simulink model "ur10_NN_v1"  (R2022b)
settings: Solver=ode4  StartTime=0.0  StopTime=5  FixedStep=0.01  MaxStep=0.1  RelTol=1e-2  AbsTol=1e-2
model workspace (MAT data in the model file):
  jointLimits = [-2.94087978961 -2.50454747661 -2.94087978961 -2.15548162621 -5.06145483078 -1.53588974176 -3.99680398707 0 0 -2.94087978961 -2.50454747661 -2.94087978961 ... (36 elements, 18x2)]
  q_points = [-0.521158884693  0.491931392418; -0.226045107026  -0.192139666701; -0.000470673510356  -0.00321781893086; 0.204187486975  0.0825184830426; -0.516935337839  0.505690245866; 0.0199734933983  0.0998802945608]
undefined symbols (not defined in the file): cbf_parms, obstacle, replay_rate, ur10
libraries: robotmaniplib x29, neural x27, robotcorelib x10
(part 2 of 2)

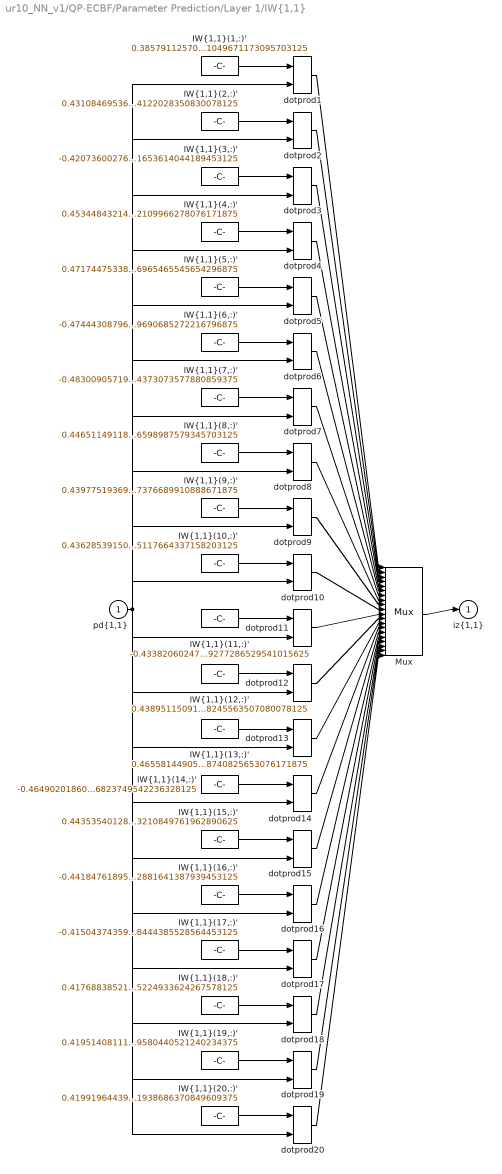
== system ur10_NN_v1/QP-ECBF/Parameter Prediction/Layer 1/IW{1,1} ==
  "pd{1,1}" : Inport  PortDimensions=1
      mask Display: e = 0.06;c1 = [120 230 180]/255;c2 = ([120 230 180]+0)/(256+128);c3 = ([120 230 180]+128)/(256+128);patch([0 1 1 0],[0 0 1 1],c1);patch([0 1 1 1-e 1-e 0+e],[0 0 1 1-e 0+e 0+e],c2);patch([0 0 1 1-e 0+e 0+e],[0 1 1 1-e 1-e 0+e],c3);plot([0 1 1 0 0],[0 0 1 1 0]);
  "IW{1,1}(1,:)'" : Constant  Value=0.385791125708176363406920472698402591049671173095703125
      mask Display: e = 0.06;c1 = [120 150 230]/255;c2 = ([120 150 230]+0)/383;c3 = ([120 150 230]+128)/383;patch([0 1 1 0],[0 0 1 1],c1);patch([0 1 1 1-e 1-e 0+e],[0 0 1 1-e 0+e 0+e],c2);patch([0 0 1 1-e 0+e 0+e],[0 1 1 1-e 1-e 0+e],c3);plot([0 1 1 0 0],[0 0 1 1 0]);disp('Weights');
  "IW{1,1}(10,:)'" : Constant  Value=0.43628539150201117724492405614000745117664337158203125
      mask Display: e = 0.06;c1 = [120 150 230]/255;c2 = ([120 150 230]+0)/383;c3 = ([120 150 230]+128)/383;patch([0 1 1 0],[0 0 1 1],c1);patch([0 1 1 1-e 1-e 0+e],[0 0 1 1-e 0+e 0+e],c2);patch([0 0 1 1-e 0+e 0+e],[0 1 1 1-e 1-e 0+e],c3);plot([0 1 1 0 0],[0 0 1 1 0]);disp('Weights');
  "IW{1,1}(11,:)'" : Constant  Value=-0.433820602471342964268075093059451319277286529541015625
      mask Display: e = 0.06;c1 = [120 150 230]/255;c2 = ([120 150 230]+0)/383;c3 = ([120 150 230]+128)/383;patch([0 1 1 0],[0 0 1 1],c1);patch([0 1 1 1-e 1-e 0+e],[0 0 1 1-e 0+e 0+e],c2);patch([0 0 1 1-e 0+e 0+e],[0 1 1 1-e 1-e 0+e],c3);plot([0 1 1 0 0],[0 0 1 1 0]);disp('Weights');
  "IW{1,1}(12,:)'" : Constant  Value=0.438951150918765187203263167248223908245563507080078125
      mask Display: e = 0.06;c1 = [120 150 230]/255;c2 = ([120 150 230]+0)/383;c3 = ([120 150 230]+128)/383;patch([0 1 1 0],[0 0 1 1],c1);patch([0 1 1 1-e 1-e 0+e],[0 0 1 1-e 0+e 0+e],c2);patch([0 0 1 1-e 0+e 0+e],[0 1 1 1-e 1-e 0+e],c3);plot([0 1 1 0 0],[0 0 1 1 0]);disp('Weights');
  "IW{1,1}(13,:)'" : Constant  Value=0.465581449051758411439294604861061088740825653076171875
      mask Display: e = 0.06;c1 = [120 150 230]/255;c2 = ([120 150 230]+0)/383;c3 = ([120 150 230]+128)/383;patch([0 1 1 0],[0 0 1 1],c1);patch([0 1 1 1-e 1-e 0+e],[0 0 1 1-e 0+e 0+e],c2);patch([0 0 1 1-e 0+e 0+e],[0 1 1 1-e 1-e 0+e],c3);plot([0 1 1 0 0],[0 0 1 1 0]);disp('Weights');
  "IW{1,1}(14,:)'" : Constant  Value=-0.464902018604204159135662166590918786823749542236328125
      mask Display: e = 0.06;c1 = [120 150 230]/255;c2 = ([120 150 230]+0)/383;c3 = ([120 150 230]+128)/383;patch([0 1 1 0],[0 0 1 1],c1);patch([0 1 1 1-e 1-e 0+e],[0 0 1 1-e 0+e 0+e],c2);patch([0 0 1 1-e 0+e 0+e],[0 1 1 1-e 1-e 0+e],c3);plot([0 1 1 0 0],[0 0 1 1 0]);disp('Weights');
  "IW{1,1}(15,:)'" : Constant  Value=0.44353540128859325619714581989683210849761962890625
      mask Display: e = 0.06;c1 = [120 150 230]/255;c2 = ([120 150 230]+0)/383;c3 = ([120 150 230]+128)/383;patch([0 1 1 0],[0 0 1 1],c1);patch([0 1 1 1-e 1-e 0+e],[0 0 1 1-e 0+e 0+e],c2);patch([0 0 1 1-e 0+e 0+e],[0 1 1 1-e 1-e 0+e],c3);plot([0 1 1 0 0],[0 0 1 1 0]);disp('Weights');
  "IW{1,1}(16,:)'" : Constant  Value=-0.441847618958016330470428556509432382881641387939453125
      mask Display: e = 0.06;c1 = [120 150 230]/255;c2 = ([120 150 230]+0)/383;c3 = ([120 150 230]+128)/383;patch([0 1 1 0],[0 0 1 1],c1);patch([0 1 1 1-e 1-e 0+e],[0 0 1 1-e 0+e 0+e],c2);patch([0 0 1 1-e 0+e 0+e],[0 1 1 1-e 1-e 0+e],c3);plot([0 1 1 0 0],[0 0 1 1 0]);disp('Weights');
  "IW{1,1}(17,:)'" : Constant  Value=-0.41504374359596785115655848130700178444385528564453125
      mask Display: e = 0.06;c1 = [120 150 230]/255;c2 = ([120 150 230]+0)/383;c3 = ([120 150 230]+128)/383;patch([0 1 1 0],[0 0 1 1],c1);patch([0 1 1 1-e 1-e 0+e],[0 0 1 1-e 0+e 0+e],c2);patch([0 0 1 1-e 0+e 0+e],[0 1 1 1-e 1-e 0+e],c3);plot([0 1 1 0 0],[0 0 1 1 0]);disp('Weights');
  "IW{1,1}(18,:)'" : Constant  Value=0.417688385219415814209042991933529265224933624267578125
      mask Display: e = 0.06;c1 = [120 150 230]/255;c2 = ([120 150 230]+0)/383;c3 = ([120 150 230]+128)/383;patch([0 1 1 0],[0 0 1 1],c1);patch([0 1 1 1-e 1-e 0+e],[0 0 1 1-e 0+e 0+e],c2);patch([0 0 1 1-e 0+e 0+e],[0 1 1 1-e 1-e 0+e],c3);plot([0 1 1 0 0],[0 0 1 1 0]);disp('Weights');
  "IW{1,1}(19,:)'" : Constant  Value=0.41951408111363386321812640744610689580440521240234375
      mask Display: e = 0.06;c1 = [120 150 230]/255;c2 = ([120 150 230]+0)/383;c3 = ([120 150 230]+128)/383;patch([0 1 1 0],[0 0 1 1],c1);patch([0 1 1 1-e 1-e 0+e],[0 0 1 1-e 0+e 0+e],c2);patch([0 0 1 1-e 0+e 0+e],[0 1 1 1-e 1-e 0+e],c3);plot([0 1 1 0 0],[0 0 1 1 0]);disp('Weights');
  "IW{1,1}(2,:)'" : Constant  Value=0.431084695364223613456289285750244744122028350830078125
      mask Display: e = 0.06;c1 = [120 150 230]/255;c2 = ([120 150 230]+0)/383;c3 = ([120 150 230]+128)/383;patch([0 1 1 0],[0 0 1 1],c1);patch([0 1 1 1-e 1-e 0+e],[0 0 1 1-e 0+e 0+e],c2);patch([0 0 1 1-e 0+e 0+e],[0 1 1 1-e 1-e 0+e],c3);plot([0 1 1 0 0],[0 0 1 1 0]);disp('Weights');
  "IW{1,1}(20,:)'" : Constant  Value=0.41991964439801332531487787491641938686370849609375
      mask Display: e = 0.06;c1 = [120 150 230]/255;c2 = ([120 150 230]+0)/383;c3 = ([120 150 230]+128)/383;patch([0 1 1 0],[0 0 1 1],c1);patch([0 1 1 1-e 1-e 0+e],[0 0 1 1-e 0+e 0+e],c2);patch([0 0 1 1-e 0+e 0+e],[0 1 1 1-e 1-e 0+e],c3);plot([0 1 1 0 0],[0 0 1 1 0]);disp('Weights');
  "IW{1,1}(3,:)'" : Constant  Value=-0.4207360027662521151370356164989061653614044189453125
      mask Display: e = 0.06;c1 = [120 150 230]/255;c2 = ([120 150 230]+0)/383;c3 = ([120 150 230]+128)/383;patch([0 1 1 0],[0 0 1 1],c1);patch([0 1 1 1-e 1-e 0+e],[0 0 1 1-e 0+e 0+e],c2);patch([0 0 1 1-e 0+e 0+e],[0 1 1 1-e 1-e 0+e],c3);plot([0 1 1 0 0],[0 0 1 1 0]);disp('Weights');
  "IW{1,1}(4,:)'" : Constant  Value=0.4534484321497032066616839074413292109966278076171875
      mask Display: e = 0.06;c1 = [120 150 230]/255;c2 = ([120 150 230]+0)/383;c3 = ([120 150 230]+128)/383;patch([0 1 1 0],[0 0 1 1],c1);patch([0 1 1 1-e 1-e 0+e],[0 0 1 1-e 0+e 0+e],c2);patch([0 0 1 1-e 0+e 0+e],[0 1 1 1-e 1-e 0+e],c3);plot([0 1 1 0 0],[0 0 1 1 0]);disp('Weights');
  "IW{1,1}(5,:)'" : Constant  Value=0.471744753381412695869556728212046436965465545654296875
      mask Display: e = 0.06;c1 = [120 150 230]/255;c2 = ([120 150 230]+0)/383;c3 = ([120 150 230]+128)/383;patch([0 1 1 0],[0 0 1 1],c1);patch([0 1 1 1-e 1-e 0+e],[0 0 1 1-e 0+e 0+e],c2);patch([0 0 1 1-e 0+e 0+e],[0 1 1 1-e 1-e 0+e],c3);plot([0 1 1 0 0],[0 0 1 1 0]);disp('Weights');
  "IW{1,1}(6,:)'" : Constant  Value=-0.474443087961794407458882005812483839690685272216796875
      mask Display: e = 0.06;c1 = [120 150 230]/255;c2 = ([120 150 230]+0)/383;c3 = ([120 150 230]+128)/383;patch([0 1 1 0],[0 0 1 1],c1);patch([0 1 1 1-e 1-e 0+e],[0 0 1 1-e 0+e 0+e],c2);patch([0 0 1 1-e 0+e 0+e],[0 1 1 1-e 1-e 0+e],c3);plot([0 1 1 0 0],[0 0 1 1 0]);disp('Weights');
  "IW{1,1}(7,:)'" : Constant  Value=-0.483009057197872238020863733254373073577880859375
      mask Display: e = 0.06;c1 = [120 150 230]/255;c2 = ([120 150 230]+0)/383;c3 = ([120 150 230]+128)/383;patch([0 1 1 0],[0 0 1 1],c1);patch([0 1 1 1-e 1-e 0+e],[0 0 1 1-e 0+e 0+e],c2);patch([0 0 1 1-e 0+e 0+e],[0 1 1 1-e 1-e 0+e],c3);plot([0 1 1 0 0],[0 0 1 1 0]);disp('Weights');
  "IW{1,1}(8,:)'" : Constant  Value=0.446511491183943232119446520300698466598987579345703125
      mask Display: e = 0.06;c1 = [120 150 230]/255;c2 = ([120 150 230]+0)/383;c3 = ([120 150 230]+128)/383;patch([0 1 1 0],[0 0 1 1],c1);patch([0 1 1 1-e 1-e 0+e],[0 0 1 1-e 0+e 0+e],c2);patch([0 0 1 1-e 0+e 0+e],[0 1 1 1-e 1-e 0+e],c3);plot([0 1 1 0 0],[0 0 1 1 0]);disp('Weights');
  "IW{1,1}(9,:)'" : Constant  Value=0.4397751936978948616996376586030237376689910888671875
      mask Display: e = 0.06;c1 = [120 150 230]/255;c2 = ([120 150 230]+0)/383;c3 = ([120 150 230]+128)/383;patch([0 1 1 0],[0 0 1 1],c1);patch([0 1 1 1-e 1-e 0+e],[0 0 1 1-e 0+e 0+e],c2);patch([0 0 1 1-e 0+e 0+e],[0 1 1 1-e 1-e 0+e],c3);plot([0 1 1 0 0],[0 0 1 1 0]);disp('Weights');
  Mux : Mux  Inputs=20
      mask Display: e = 0.06;c1 = [120 150 230]/255;c2 = ([120 150 230]+0)/383;c3 = ([120 150 230]+128)/383;patch([0 1 1 0],[0 0 1 1],c1);patch([0 1 1 1-e 1-e 0+e],[0 0 1 1-e 0+e 0+e],c2);patch([0 0 1 1-e 0+e 0+e],[0 1 1 1-e 1-e 0+e],c3);plot([0 1 1 0 0],[0 0 1 1 0]);disp('Mux');
  dotprod{1..20} (20 alike) : neural/Weight Functions/dotprod
  "iz{1,1}" : Outport
      mask Display: e = 0.06;c1 = [120 230 180]/255;c2 = ([120 230 180]+0)/(256+128);c3 = ([120 230 180]+128)/(256+128);patch([0 1 1 0],[0 0 1 1],c1);patch([0 1 1 1-e 1-e 0+e],[0 0 1 1-e 0+e 0+e],c2);patch([0 0 1 1-e 0+e 0+e],[0 1 1 1-e 1-e 0+e],c3);plot([0 1 1 0 0],[0 0 1 1 0]);
  wires:
  "IW{1,1}(1,:)'"/1 -> dotprod1/1
  "pd{1,1}"/1 -> dotprod1/2, dotprod2/2, dotprod3/2, dotprod4/2, dotprod5/2, dotprod6/2, dotprod7/2, dotprod8/2, dotprod9/2, dotprod10/2, dotprod11/2, dotprod12/2, dotprod13/2, dotprod14/2, dotprod15/2, dotprod16/2, dotprod17/2, dotprod18/2, dotprod19/2, dotprod20/2
  dotprod1/1 -> Mux/1
  "IW{1,1}(2,:)'"/1 -> dotprod2/1
  dotprod2/1 -> Mux/2
  "IW{1,1}(3,:)'"/1 -> dotprod3/1
  dotprod3/1 -> Mux/3
  "IW{1,1}(4,:)'"/1 -> dotprod4/1
  dotprod4/1 -> Mux/4
  "IW{1,1}(5,:)'"/1 -> dotprod5/1
  dotprod5/1 -> Mux/5
  "IW{1,1}(6,:)'"/1 -> dotprod6/1
  dotprod6/1 -> Mux/6
  "IW{1,1}(7,:)'"/1 -> dotprod7/1
  dotprod7/1 -> Mux/7
  "IW{1,1}(8,:)'"/1 -> dotprod8/1
  dotprod8/1 -> Mux/8
  "IW{1,1}(9,:)'"/1 -> dotprod9/1
  dotprod9/1 -> Mux/9
  "IW{1,1}(10,:)'"/1 -> dotprod10/1
  dotprod10/1 -> Mux/10
  "IW{1,1}(11,:)'"/1 -> dotprod11/1
  dotprod11/1 -> Mux/11
  "IW{1,1}(12,:)'"/1 -> dotprod12/1
  dotprod12/1 -> Mux/12
  "IW{1,1}(13,:)'"/1 -> dotprod13/1
  dotprod13/1 -> Mux/13
  "IW{1,1}(14,:)'"/1 -> dotprod14/1
  dotprod14/1 -> Mux/14
  "IW{1,1}(15,:)'"/1 -> dotprod15/1
  dotprod15/1 -> Mux/15
  "IW{1,1}(16,:)'"/1 -> dotprod16/1
  dotprod16/1 -> Mux/16
  "IW{1,1}(17,:)'"/1 -> dotprod17/1
  dotprod17/1 -> Mux/17
  "IW{1,1}(18,:)'"/1 -> dotprod18/1
  dotprod18/1 -> Mux/18
  "IW{1,1}(19,:)'"/1 -> dotprod19/1
  dotprod19/1 -> Mux/19
  "IW{1,1}(20,:)'"/1 -> dotprod20/1
  dotprod20/1 -> Mux/20
  Mux/1 -> "iz{1,1}"/1

== system ur10_NN_v1/QP-ECBF/Parameter Prediction/Layer 2/Delays 1 ==
  "p{2}" : Inport  PortDimensions=20
      mask Display: e = 0.06;c1 = [120 230 180]/255;c2 = ([120 230 180]+0)/(256+128);c3 = ([120 230 180]+128)/(256+128);patch([0 1 1 0],[0 0 1 1],c1);patch([0 1 1 1-e 1-e 0+e],[0 0 1 1-e 0+e 0+e],c2);patch([0 0 1 1-e 0+e 0+e],[0 1 1 1-e 1-e 0+e],c3);plot([0 1 1 0 0],[0 0 1 1 0]);
  mux : Mux  Inputs=1
      mask Display: e = 0.06;c1 = [120 150 230]/255;c2 = ([120 150 230]+0)/383;c3 = ([120 150 230]+128)/383;patch([0 1 1 0],[0 0 1 1],c1);patch([0 1 1 1-e 1-e 0+e],[0 0 1 1-e 0+e 0+e],c2);patch([0 0 1 1-e 0+e 0+e],[0 1 1 1-e 1-e 0+e],c3);plot([0 1 1 0 0],[0 0 1 1 0]);disp('Mux')
  "pd{2,1}" : Outport
      mask Display: e = 0.06;c1 = [120 230 180]/255;c2 = ([120 230 180]+0)/(256+128);c3 = ([120 230 180]+128)/(256+128);patch([0 1 1 0],[0 0 1 1],c1);patch([0 1 1 1-e 1-e 0+e],[0 0 1 1-e 0+e 0+e],c2);patch([0 0 1 1-e 0+e 0+e],[0 1 1 1-e 1-e 0+e],c3);plot([0 1 1 0 0],[0 0 1 1 0]);
  wires:
  "p{2}"/1 -> mux/1
  mux/1 -> "pd{2,1}"/1

== system ur10_NN_v1/QP-ECBF/Parameter Prediction/Layer 2/LW{2,1} ==
  "ad{2,1}" : Inport  PortDimensions=20
      mask Display: e = 0.06;c1 = [120 230 180]/255;c2 = ([120 230 180]+0)/(256+128);c3 = ([120 230 180]+128)/(256+128);patch([0 1 1 0],[0 0 1 1],c1);patch([0 1 1 1-e 1-e 0+e],[0 0 1 1-e 0+e 0+e],c2);patch([0 0 1 1-e 0+e 0+e],[0 1 1 1-e 1-e 0+e],c3);plot([0 1 1 0 0],[0 0 1 1 0]);
  "IW{2,1}(1,:)'" : Constant  Value=[-0.1626878657231537184113534522111876867711544036865234375;-0.1200341041433554689632501322194002568721771240234375;0.1005644547301407787376348323959973640739917755126953125;-0.0218554638658896051295332796371440053917467594146728515625;0.046984730038880005709156506554791121743619441986083984375;-0.06521551214731112489086939376647933386266231536865234375;-0.09351088155010280067447325791363255120813846588134765625;0.054747137380286116370431415134589769877493381500244140625;0.035620000191153682045364092800809885375201702117919921875;0.00647129243408957333105746556611848063766956329345703125;0.0304926056112096548200707246678575756959617137908935546875;-0.032706609699335316421286989907457609660923480987548828125;-0.03896160134336344726957435113945393823087215423583984375;0.0120722770013152007340107019217612105421721935272216796875;0.0089858125649034288617844623558994499035179615020751953125;-0.0185507146410883345943876321371135418303310871124267578125;-0.01055971666121561895745895043319251271896064281463623046875;0.0011611856964841254895304256677945886622183024883270263671875;0.021181318555724769348014291381332441233098506927490234375;0.0093270870010835615904198903081123717129230499267578125]
      mask Display: e = 0.06;c1 = [120 150 230]/255;c2 = ([120 150 230]+0)/383;c3 = ([120 150 230]+128)/383;patch([0 1 1 0],[0 0 1 1],c1);patch([0 1 1 1-e 1-e 0+e],[0 0 1 1-e 0+e 0+e],c2);patch([0 0 1 1-e 0+e 0+e],[0 1 1 1-e 1-e 0+e],c3);plot([0 1 1 0 0],[0 0 1 1 0]);disp('weights');
  "IW{2,1}(2,:)'" : Constant  Value=[0.00756061639430020450414193788901684456504881381988525390625;0.08750502387805585147173559334987658075988292694091796875;-0.07664562041841531392361019925374421291053295135498046875;0.098644587802629579709190466019208543002605438232421875;0.0880836660792229941829845074607874266803264617919921875;-0.103339761351128045507863362217904068529605865478515625;-0.08880949371971062766828453050038660876452922821044921875;0.0535830427909179396461780697791255079209804534912109375;0.0159742324232805925354750087308275396935641765594482421875;-0.0261153336850302696114933809212743653915822505950927734375;0.036032274140479401969283657081177807413041591644287109375;-0.04867981331125814659088746338966302573680877685546875;-0.0776917850793362452233026260728365741670131683349609375;0.0769932486910005764446651710386504419147968292236328125;-0.0472688243128740470666571127367205917835235595703125;0.041077261467079788370693194110572221688926219940185546875;-0.00795559040924911052561352420298135257326066493988037109375;0.0177287962921194065801788752878564991988241672515869140625;0.0268925673466994530347307090778485871851444244384765625;0.04768874943697347379423234770001727156341075897216796875]
      mask Display: e = 0.06;c1 = [120 150 230]/255;c2 = ([120 150 230]+0)/383;c3 = ([120 150 230]+128)/383;patch([0 1 1 0],[0 0 1 1],c1);patch([0 1 1 1-e 1-e 0+e],[0 0 1 1-e 0+e 0+e],c2);patch([0 0 1 1-e 0+e 0+e],[0 1 1 1-e 1-e 0+e],c3);plot([0 1 1 0 0],[0 0 1 1 0]);disp('weights');
  Mux : Mux  Inputs=2
      mask Display: e = 0.06;c1 = [120 150 230]/255;c2 = ([120 150 230]+0)/383;c3 = ([120 150 230]+128)/383;patch([0 1 1 0],[0 0 1 1],c1);patch([0 1 1 1-e 1-e 0+e],[0 0 1 1-e 0+e 0+e],c2);patch([0 0 1 1-e 0+e 0+e],[0 1 1 1-e 1-e 0+e],c3);plot([0 1 1 0 0],[0 0 1 1 0]);disp('Mux');
  dotprod1 : neural/Weight Functions/dotprod
  dotprod2 : neural/Weight Functions/dotprod
  "lz{2,1}" : Outport
      mask Display: e = 0.06;c1 = [120 230 180]/255;c2 = ([120 230 180]+0)/(256+128);c3 = ([120 230 180]+128)/(256+128);patch([0 1 1 0],[0 0 1 1],c1);patch([0 1 1 1-e 1-e 0+e],[0 0 1 1-e 0+e 0+e],c2);patch([0 0 1 1-e 0+e 0+e],[0 1 1 1-e 1-e 0+e],c3);plot([0 1 1 0 0],[0 0 1 1 0]);
  wires:
  "IW{2,1}(1,:)'"/1 -> dotprod1/1
  "ad{2,1}"/1 -> dotprod1/2, dotprod2/2
  dotprod1/1 -> Mux/1
  "IW{2,1}(2,:)'"/1 -> dotprod2/1
  dotprod2/1 -> Mux/2
  Mux/1 -> "lz{2,1}"/1

== matlab function ur10_NN_v1/DISPLAYS/MATLAB Function ==
  data: t input; y1 output; y2 output; y3 output; obs input
function [y1,y2,y3] = fcn(t, obs)
    center = [obs(1) ; obs(2) ; obs(3)];
    radius = obs(4);
    theta = t*1*(2*pi/2.5)-(pi/2);
    traj1 = center + radius*[   0*ones(size(theta));    cos(theta);             sin(theta)              ];
    traj2 = center + radius*[   sin(theta);             0*ones(size(theta));    cos(theta)              ];
    traj3 = center + radius*[   cos(theta);             sin(theta);             0*ones(size(theta))     ];

       
    y1 = traj1;
    y2 = traj2;
    y3 = traj3;

== matlab function ur10_NN_v1/QP-ECBF/Closest Joint Selection1/MATLAB Function ==
  data: obs input; ee_pos input; w3_pos input; w2_pos input; eta_pos output; w1_pos input; Jclose output; test2 output; J input
function [eta_pos, Jclose, test2] = fcn(obs, ee_pos, w3_pos, w2_pos, w1_pos, J)

    j_pos       = [ ee_pos' ; w3_pos' ; w2_pos' ; w1_pos' ] ;
    
    min_sep     = 10000;
    min_joint   = 0;
    
    for i = 1:4
        
        sep_dist = sqrt( (obs(1) - j_pos(i,1))^2 + (obs(2) - j_pos(i,2))^2 + (obs(3) - j_pos(i,3))^2 ) - obs(4);
        
        if sep_dist < min_sep
            min_sep = sep_dist;
            min_joint = i;
        end
    end



%% Function Outputs
eta_pos     = j_pos(min_joint,:);
Jclose      = J(:,:,min_joint);
test2       = [min_sep ; min_joint];

== matlab function ur10_NN_v1/QP-ECBF/eCBF-QP ==
  settings: updateMethod=DISCRETE
  data: u_nom input; X1 input; X2 input; M input; u output; G input; C input; flag_qp output; test2 output; J6 input; Jd_qd6 input; obs input; cbf_parms input
function [u, flag_qp, test2]       = fcn(u_nom,X1, X2, M, G, C, J6, Jd_qd6, obs, cbf_parms)
    
    % Select position elements from jacobian inputs (bottom half rows 4:6)
    
    J           = J6(4:6,:);    % J will refer to position elments of J6
    Jd_qd       = Jd_qd6(4:6,:);

    % end effector states 
    %world frame positions
    x_pos       = X1(4);
    y_pos       = X1(5);
    z_pos       = X1(6);
    x_eul       = X1(1);
    y_eul       = X1(2);
    z_eul       = X1(3);
        
    %world frame velocities
    x_vel       = X2(4);
    y_vel       = X2(5);
    z_vel       = X2(6);
    x_wvel      = X2(1);
    y_wvel      = X2(2);
    z_wvel      = X2(3);
    
    eta_dot     = [ x_vel ; y_vel ; z_vel ]; % velocity column vector used for Lfh
    
    %Obstacle info
    r_obs       = obs(4);
    x_obs       = obs(1);
    y_obs       = obs(2);
    z_obs       = obs(3);
    
    % Variables used in ECBF
    m           = inv(M);
    CDG         = C + G;    % no damping in model yet!
    
    sep_x       = x_pos - x_obs;
    sep_y       = y_pos - y_obs;
    sep_z       = z_pos - z_obs;


    r_body      = 0.1;
    
    sep_dist    = sqrt( sep_x^2 + sep_y^2 + sep_z^2) - r_obs - r_body;
        
    %CBF parameters
    % changed to input variable cbf_parms = [ k1, k2, rpad ]
    k1          = cbf_parms(1);
    k2          = cbf_parms(2);
    r_pad       = cbf_parms(3);
    
    Sn          = [ 2*sep_x , 2*sep_y , 2*sep_z ];    % 1x3
    
    h           = (sep_x^2) + (sep_y^2) + (sep_z^2) - r_pad^2 - r_body^2 - r_obs^2;
    Lfh         = Sn*eta_dot;   %2*a*sep_x*x_vel + 2*b*sep_y*y_vel + 2*c*sep_z*z_vel;
    
    L2fh_nom    = 2*x_vel^2 + 2*y_vel^2 + 2*z_vel^2 ...
                  + Sn*Jd_qd ...
                  + Sn*(J*(m*(u_nom - CDG)));
 
    % quadprog parameters
  
    H       = 2*diag(ones(6,1));
    f       = zeros(6,1); 
    
    %                      A            x
    %             ==================   ----
    %  Ax < b   : Sn   *   J   *   m * u_qp    ...
    %             1x3     3x6     6x6  6x1 
    %
    
    A       = Sn*J*m;
    b       = L2fh_nom + k2*Lfh + k1*h; 
    
    Aeq     = [ 0 0 0 0 0 1 ;
                0 0 0 0 1 0 ;
                0 0 0 1 0 0 ];
    
    beq     = [ 0 ;    % needs same number rows as Aeq
                0 ;
                0 ];
       
    flag    = 0;
    u_qp    = zeros(6,1);
    
    coder.extrinsic('quadprog');
    
    options             = optimset('Display', 'off'); % set off to supress quadprog messages (faster)
    [output, ~, flag]   = quadprog(H,f,A,b,Aeq,beq,[],[],[],options);

    if flag == 1
        u_qp   = output;
    else
        u_qp   = zeros(6,1);
    end
    
    %% Function outputs
    flag_qp     = flag;
    test2       = sep_dist;
    u           = u_qp;
